simulink subsystem "Vehicle_Dynamics_2"  (R2025b)
settings: Solver=VariableStepAuto  StartTime=0.0  StopTime=10.0  RelTol=1e-3
undefined symbols (not defined in the file): J_d, MaxMdot_d, TB_d
settings Model: Creator=pplat  LastModifiedBy=pplat

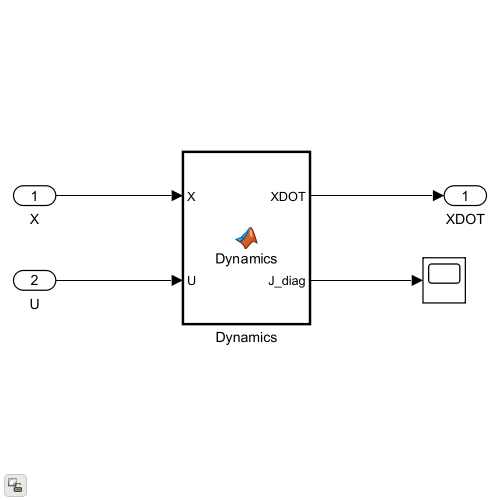
[thumbnail: Simulink's stored preview of the top-level diagram]
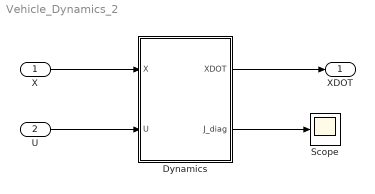
== system Vehicle_Dynamics_2 ==
  X : Inport  PortDimensions=[15,1]
  U : Inport  Port=2  PortDimensions=[4,1]
  Dynamics : MATLAB Function  TreatAsAtomicUnit=on
  Scope : Scope
      settings: ActiveDisplayYMinimum=6.4296735269491379  ActiveDisplayYMaximum=93.684040043646021  DataLoggingVariableName=ScopeData14
  XDOT : Outport
  wires:
  U/1 -> Dynamics/2(U)
  X/1 -> Dynamics/1(X)
  Dynamics/2(J_diag) -> Scope/1
  Dynamics/1(XDOT) -> XDOT/1

== matlab function Vehicle_Dynamics_2/Dynamics ==
  data: X input; XDOT output; U input; J_d parameter; TB_d parameter; J_diag output; MaxMdot_d parameter
function [XDOT, J_diag] = Dynamics(X, U, J_d, TB_d, MaxMdot_d)
[XDOT, J_diag] = TOAD_Dynamics(X, U, J_d, TB_d, MaxMdot_d);
